simulink model "EMPlanner_cs_old"  (R2020a)
settings: Solver=ode5  StartTime=0.0  StopTime=55  FixedStep=1/1000  RelTol=1e-3
PreLoadFcn:
  | mbxruntime.callbacks.PreLoadFcn(bdroot);
PostLoadFcn:
  | mbxruntime.callbacks.PostLoadFcn(bdroot);
InitFcn:
  | mbxruntime.callbacks.InitFcn(bdroot);
StartFcn:
  | mbxruntime.callbacks.StartFcn(bdroot);
StopFcn:
  | mbxruntime.callbacks.StopFcn(bdroot);
model workspace: external: MAT-File .\EMPlanner_cs_hws.mat (data not in the file)
values from neighbouring files (symbols this model uses):
  c_factor = 43.75    [emplanner_init.m]
  cf = -175016    [emplanner_init.m]
  cr = -130634    [emplanner_init.m]
  KD_PID_distance = 0.0    (= 0)    [emplanner_init.m]
  KD_PID_speed = 0    [emplanner_init.m]
  KI_PID_distance = 0.0    (= 0)    [emplanner_init.m]
  KI_PID_speed = 0    [emplanner_init.m]
  KP_PID_distance = 0.5    [emplanner_init.m]
  KP_PID_speed = 1.8    [emplanner_init.m]
  la = 1.265    [emplanner_init.m]
  lb = 2.947-1.265    (= 1.682)    [emplanner_init.m]
  LQR_K1 = k(:,1)'    [emplanner_init.m]
  LQR_K2 = k(:,2)'    [emplanner_init.m]
  LQR_K3 = k(:,3)'    [emplanner_init.m]
  LQR_K4 = k(:,4)'    [emplanner_init.m]
  m = 2020    [emplanner_init.m]
  path_x = [7.7742 8.77358225507 9.77170536558 10.7685522493 11.7641171228 12.7583983581 13.7513958557 14.7431100776 15.7335416918 16.7226914411 17.7105600952 18.6971484329 ... (551 elements, 551x1)]    [test_path.mat]
  path_y = [-207.8202 -207.82020006 -207.820200616 -207.820202023 -207.82020429 -207.820207237 -207.820210603 -207.820214131 -207.82021762 -207.820220941 -207.820224011 -207.820226778 ... (551 elements, 551x1)]    [test_path.mat]
  rack_displacement = [-39.14 , -37.2 , -35.29 , -33.43 , -31.6 , -29.81 , -28.06 , -26.34 , -24.66 ,      -23.01 , -21.38 , -19.79 , -18.23 , -16.69 , -15.18 , -13.7 , -12.23 , -10.8 , -9.38 , -7.98 ,     -6.61 , -5.25 , -3.91 , -2.59 , -1.29 , 0 , 1.27 , 2.54 , 3.78 , 5.02 , 6.24 , 7.46 , 8.66 ,      9.86 , 11.05 , 12.24 , 13.41 , 14.59 , 15.76 , 16.92 , 18.09 , 19.25 , 20.42 , 21.59 , 22.76 ,      23.93 , 25.11 , 26 ...(+26 chars)    [emplanner_init.m]
  right_wheel_ground = [-70 ,-67.2 , -64.4 , -61.6 , -58.8 , -56 , -53.2 , -50.4 , -47.6 , -44.8 , -42 ,      -39.2 , -36.4 , -33.6 , -30.8 , -28 , -25.2 , -22.4 , -19.6 , -16.8 , -14 , -11.2 , -8.4 , -5.6 ,      -2.8 , 0 , 2.8 , 5.6 , 8.4 , 11.2 , 14 , 16.8 , 19.6 , 22.4 , 25.2 , 28 , 30.8 , 33.6 , 36.4 ,      39.2 , 42 , 44.8 , 47.6 , 50.4 , 53.2 , 56 , 58.8 , 61.6 , 64.4 , 67.2 , 70 ]    [emplanner_init.m]
  vx_break_point = zeros(1,5000)    [emplanner_init.m]
undefined symbols (not defined in the file or in its folder): aubr, DiscIntNeverNeededParam, tablebr, vubr, warningInitialVelocity, x0
libraries: simulink x19, PreScanSimulinkLibrary x10, simulink_extras x5, Solver_SF x1
(part 7 of 8)

== matlab function EMPlanner_cs_old/Audi_A8_Sedan_1/decision&planning module/EM Planner/calc plan start info and stitch trajectory1 ==
  data: pre_trajectory_x input; plan_start_x output; pre_trajectory_y input; pre_trajectory_heading input; pre_trajectory_kappa input; pre_trajectory_velocity input; pre_trajectory_accel input; pre_trajectory_time input; current_time input; host_x input; host_y input; host_heading_xy input; host_vx input; host_vy input; host_ax input; host_ay input; plan_start_y output; plan_start_heading output; plan_start_kappa output; plan_start_vx output; plan_start_vy output; plan_start_ax output; plan_start_ay output; plan_start_time output; stitch_x output; stitch_y output; stitch_heading output; stitch_kappa output; stitch_speed output; stitch_accel output; stitch_time output
function [plan_start_x,plan_start_y,plan_start_heading,plan_start_kappa,plan_start_vx,plan_start_vy,plan_start_ax,...
    plan_start_ay,plan_start_time,stitch_x,stitch_y,stitch_heading,stitch_kappa,stitch_speed,stitch_accel,stitch_time] ...
    = fcn(pre_trajectory_x,pre_trajectory_y,pre_trajectory_heading,pre_trajectory_kappa,pre_trajectory_velocity,...
    pre_trajectory_accel,pre_trajectory_time,current_time,host_x,host_y,host_heading_xy,host_vx,host_vy,host_ax,host_ay)
%该函数将计算规划的起点以及拼接轨迹的信息
%输入 上一周期的规划结果信息pre_trajectory x ,y,heading,kappa,velocity,accel,time
%     本周期的绝对时间current_time
%     定位信息host x,y,heading,kappa,vx,vy,ax,ay
%输出 规划起点信息plan_start x,y,heading,kappa,vx,vy,ax,ay(vx,vy,ax,ay)是世界坐标系的
%     待拼接的轨迹信息，一般在上一周期的轨迹中的current_time+100ms，往前取20个点。
%     当规划完成后，本周期的规划结果和stitch_trajectory一起拼好发给控制

%输出初始化
stitch_x = zeros(20,1);
stitch_y = zeros(20,1);
stitch_heading = zeros(20,1);
stitch_kappa = zeros(20,1);
stitch_speed = zeros(20,1);
stitch_accel = zeros(20,1);
%时间为负代表没有对应的拼接轨迹
stitch_time = ones(20,1)*-1;

%申明全局变量
persistent is_first_run;
if isempty(is_first_run)
    %代表代码首次运行
    is_first_run = 0;
    %按照轨迹拼接算法，应该用车辆动力学递推，但是首次运行车辆的速度都是0，所以没必要递推了
    plan_start_x = host_x;
    plan_start_y = host_y;
    plan_start_heading = host_heading_xy;
    plan_start_kappa = 0;
    plan_start_vx = 0;
    plan_start_vy = 0;
    plan_start_ax = 0;
    plan_start_ay = 0;
    %规划的起点的时间应该是当前时间+100ms
    plan_start_time = current_time + 0.1;
else
    %该函数不是首次运行
    x_cur = host_x;
    y_cur = host_y;
    heading_cur = host_heading_xy;
    kappa_cur = 0;
    %vx vy ax ay要转换成世界坐标系
    vx_cur = host_vx*cos(heading_cur) - host_vy*sin(heading_cur);
    vy_cur = host_vx*sin(heading_cur) + host_vy*cos(heading_cur);
    ax_cur = host_ax*cos(heading_cur) - host_ay*sin(heading_cur);
    ay_cur = host_ax*sin(heading_cur) + host_ay*cos(heading_cur);
    %规划周期
    dt = 0.1;
    %由于不是首次运行了，有上一时刻的轨迹了，找到上一周期轨迹规划的本周期车辆应该在的位置
    for i = 1:length(pre_trajectory_time) - 1
        if (pre_trajectory_time(i) <= current_time && pre_trajectory_time(i + 1) > current_time)
            break;
        end
    end
    %上一周期规划的本周期的车应该在的位置
    pre_x_desire = pre_trajectory_x(i);
    pre_y_desire = pre_trajectory_y(i);
    pre_heading_desire = pre_trajectory_heading(i);
    %计算横纵向误差
    %切向量
    tor = [cos(pre_heading_desire);sin(pre_heading_desire)];
    %法向量
    nor = [-sin(pre_heading_desire);cos(pre_heading_desire)];
    %误差向量
    d_err = [host_x;host_y] - [pre_x_desire;pre_y_desire];
    %纵向误差
    lon_err = abs(d_err'*tor);
    %横向误差
    lat_err = abs(d_err'*nor);
    %纵向误差大于2.5 横向误差大于0.5 认为控制没跟上
    if (lon_err > 2.5)||(lat_err > 0.5)
        %此分支处理控制未跟上的情况，规划起点通过运动学递推
        plan_start_x = x_cur + vx_cur * dt + 0.5 * ax_cur * dt * dt;
        plan_start_y = y_cur + vy_cur * dt + 0.5 * ay_cur * dt * dt;
        plan_start_vx = vx_cur + ax_cur * dt;
        plan_start_vy = vy_cur + ay_cur * dt;
        plan_start_heading = atan2(plan_start_vy,plan_start_vx);
        plan_start_ax = ax_cur;
        plan_start_ay = ay_cur;
        plan_start_kappa = kappa_cur;
        plan_start_time = current_time + 0.1;
        return;
    else
        %此分支表示控制能跟的上规划，开始拼接
        for j = i:length(pre_trajectory_time) - 1
            if (pre_trajectory_time(j) <= current_time + 0.1)&&(pre_trajectory_time(j + 1) > current_time + 0.1)
                break;
            end
        end
        %注：此算法要能运行需要trajectory的点有很高的密度
        plan_start_x = pre_trajectory_x(j);
        plan_start_y = pre_trajectory_y(j);
        plan_start_heading = pre_trajectory_heading(j);
        plan_start_kappa = pre_trajectory_kappa(j);
        %这里的pre_trajectory的速度,加速度是指轨迹的切向速度，切向加速度
        plan_start_vx = pre_trajectory_velocity(j) * cos(plan_start_heading);
        plan_start_vy = pre_trajectory_velocity(j) * sin(plan_start_heading);
        %pre_trajectory的加速度是切向加速度，要想计算ax,ay还要计算法向加速度
        %计算轨迹在current_time + 100ms 这个点的切向量法向量
        tor = [cos(plan_start_heading);sin(plan_start_heading)];
        nor = [-sin(plan_start_heading);cos(plan_start_heading)];
        a_tor = pre_trajectory_accel(j) * tor;
        a_nor = pre_trajectory_velocity(j)^2 * plan_start_kappa * nor ;
        plan_start_ax = a_tor(1) + a_nor(1);
        plan_start_ay = a_tor(2) + a_nor(2);
        plan_start_time = pre_trajectory_time(j);
        %计算拼接轨迹
        %j 表示 current_time + 0.1 的时间点在 pre_trajectory_time的编号
        %拼接是往从j开始，往前拼接20个，也就是pre_trajectory(j-1),j-2,j-3,....j-19
        %分两种情况，如果j小于20，意味着前面的轨迹点不够20个
        %如果j >= 20,意味着前面的点多于20个
        %还有一个细节需要考虑，pre_trajectory x(j) y(j) ....是规划的起点，那么在轨迹拼接时
        %需不需要在stitch_trajectory中把pre_trajectory x(j) y(j) ....包含进去
        %答案是否定的，不应该包进去，因为规划的起点会在规划模块计算完成后的结果中包含，如果在拼接的时候
        %还要包含，那就等于规划起点包含了两次
        %除非本周期计算的轨迹不包含规划起点，那么stitch_trajectory可以包含规划起点。
        %如果本周期计算的轨迹包含规划起点，那么stitch_trajectory就不可以包含规划起点。
        %我们选择规划包含起点，拼接不包含起点的做法
        
        %把起点去掉
        j = j - 1;
        if j >= 20
            stitch_x = pre_trajectory_x(j - 19:j);
            stitch_y = pre_trajectory_y(j - 19:j);
            stitch_heading = pre_trajectory_heading(j - 19:j);
            stitch_kappa = pre_trajectory_kappa(j - 19:j);
            stitch_speed = pre_trajectory_velocity(j - 19:j);
            stitch_accel = pre_trajectory_accel(j - 19:j);
            stitch_time = pre_trajectory_time(j - 19:j);
        else
            stitch_x(20 - j + 1:20) = pre_trajectory_x(1:j);
            stitch_y(20 - j + 1:20) = pre_trajectory_y(1:j);
            stitch_heading(20 - j + 1:20) = pre_trajectory_heading(1:j);
            stitch_kappa(20 - j + 1:20) = pre_trajectory_kappa(1:j);
            stitch_speed(20 - j + 1:20) = pre_trajectory_velocity(1:j);
            stitch_accel(20 - j + 1:20) = pre_trajectory_accel(1:j);
            stitch_time(20 - j + 1:20) = pre_trajectory_time(1:j);           
        end   
    end    
end

== matlab function EMPlanner_cs_old/Audi_A8_Sedan_1/decision&planning module/EM Planner/genrate index to s ==
  data: path_x_set_gcs input; matchPoint_index_s_set_fcs output; path_y_set_gcs input; path_heading_set_gcs input; origin_match_point_index input; origin_point_x_gcs input; origin_point_y_gcs input
function matchPoint_index_s_set_fcs = fun(path_x_set_gcs,path_y_set_gcs,path_heading_set_gcs,...
    origin_match_point_index,origin_point_x_gcs,origin_point_y_gcs)
% 该函数将以给定路径采样点为s轴 取自身在给定路径上投影点作为坐标原点 来求出每个采样点编号和对应s坐标的集合
% path_x_set_gcs,path_y_set_gcs 给定路径采样点集合
% origin_match_point_index,origin_point_x_gcs,origin_point_y_gcs   坐标原点信息
% 输出初始化
matchPoint_index_s_set_fcs = zeros(length(path_x_set_gcs),1);
% 首先给定路径采样点每个点到第一个采样点的弧长
for i = 2:length(path_x_set_gcs)
    dis = sqrt((path_x_set_gcs(i)-path_x_set_gcs(i-1))^2+(path_y_set_gcs(i)-path_y_set_gcs(i-1))^2); % 以直线代替相邻点弧长
    matchPoint_index_s_set_fcs(i) = dis + matchPoint_index_s_set_fcs(i-1); % 累加得到
end
%再求出坐标原点到第一个采样点的弧长
s = CalSFromOriginPoint(matchPoint_index_s_set_fcs,path_x_set_gcs,path_y_set_gcs,path_heading_set_gcs,...
                            origin_point_x_gcs,origin_point_y_gcs,origin_match_point_index);
% 得到每个采样点到坐标原点的弧长对应关系 亦即真正的s坐标对应编号关系
matchPoint_index_s_set_fcs = matchPoint_index_s_set_fcs - ones(length(path_x_set_gcs),1)*s;
end

== stateflow chart EMPlanner_cs_old/Audi_A8_Sedan_1/Chart ==
  (default) -> (junction 5)
  (junction 5) -> (junction 7)
  (junction 7) -> (junction 9) [order 1] : [i >= 100]
  (junction 7) -> (junction 13) [order 2] : {
      | i = i + 1;
      | }
  (junction 9) -> (junction 11) : {
      | do_planning;
      | i = 1;
      | }
  (junction 11) -> (junction 13)
  (junction 13) -> (junction 16)
  (junction 16) -> (junction 18) [order 1] : [j >= 10]
  (junction 16) -> (junction 22) [order 2] : {
      | j = j + 1;
      | }
  (junction 18) -> (junction 20) : {
      | do_control;
      | j = 1;
      | }
  (junction 20) -> (junction 22)
  (junction 22) -> (junction 25)
  data: i local =1; j local =1
  events: do_planning output FUNCTION_CALL_EVENT; do_control output FUNCTION_CALL_EVENT

== matlab function EMPlanner_cs_old/Audi_A8_Sedan_1/decision&planning module/EM Planner/Cartesian2Frenet/MATLAB Function3 ==
  data: l_set input; s_dot_set output; vx_set input; vy_set input; proj_heading_set input; proj_kappa_set input; l_dot_set output; dl_set output
function [s_dot_set,l_dot_set,dl_set] = fcn(l_set,vx_set,vy_set,proj_heading_set,proj_kappa_set)
%该函数将计算frenet坐标系下的s_dot, l_dot, dl/ds
n = 128;
% 输出初始化
s_dot_set = ones(n,1)*nan;
l_dot_set = ones(n,1)*nan;
dl_set = ones(n,1)*nan;

for i = 1 : length(l_set)
    if isnan(l_set(i))
        break;
    end
    v_h = [vx_set(i);vy_set(i)];
    n_r = [-sin(proj_heading_set(i));cos(proj_heading_set(i))];
    t_r = [cos(proj_heading_set(i));sin(proj_heading_set(i))];
    l_dot_set(i) = v_h'*n_r;
    s_dot_set(i) = v_h'*t_r/(1 - proj_kappa_set(i)*l_set(i));
    %%%向量法做cartesian与frenet的转换要更简单，但是也有缺点，向量法必须依赖速度加速度
    %l' = l_dot/s_dot 但是如果s_dot = 0 此方法就失效了
    if abs(s_dot_set(i)) < 1e-6
        dl_set(i) = 0;
    else
        dl_set(i) = l_dot_set(i)/s_dot_set(i);
    end
end

== matlab function EMPlanner_cs_old/Audi_A8_Sedan_1/decision&planning module/EM Planner/Cartesian2Frenet/MATLAB Function ==
  data: x_set_gcs input; s_set_fcs output; y_set_gcs input; path_x_set_gcs input; path_y_set_gcs input; path_heading_set_gcs input; match_point_index_set input; proj_point_x_set_gcs input; proj_point_y_set_gcs input; proj_point_heading_set_gcs input; l_set_fcs output; matchPoint_index_s_set_fcs input
function [s_set_fcs,l_set_fcs] = fun(x_set_gcs,y_set_gcs,path_x_set_gcs,path_y_set_gcs,path_heading_set_gcs,match_point_index_set,...
    proj_point_x_set_gcs,proj_point_y_set_gcs,proj_point_heading_set_gcs,matchPoint_index_s_set_fcs)
% 将函数批量将给定点的(x,y)转化成(s,l)
% 假设最多有181个点需要转换坐标
n = 181;
% 输出初始化
s_set_fcs = ones(n,1)*nan; l_set_fcs = ones(n,1)*nan;
for i = 1:length(x_set_gcs)
    if isnan(x_set_gcs(i))
        break;
    end
    s_set_fcs(i) = CalSFromOriginPoint(matchPoint_index_s_set_fcs,path_x_set_gcs,path_y_set_gcs,path_heading_set_gcs,...
                                proj_point_x_set_gcs(i),proj_point_y_set_gcs(i),match_point_index_set(i));
    vector_rh = [x_set_gcs(i),y_set_gcs(i)];
    vector_rp = [proj_point_x_set_gcs(i),proj_point_y_set_gcs(i)];
    vector_np = [-sin(proj_point_heading_set_gcs(i)),cos(proj_point_heading_set_gcs(i))];
    l_set_fcs(i) = dot(vector_rh-vector_rp, vector_np);
end
end

== matlab function EMPlanner_cs_old/Audi_A8_Sedan_2/PathFollower_Preview_1/LateralController/Calculate delta steering error/eml_delta_steering_error ==
  data: v_x_vehicle input; v_x_vehicle_Min input; t_Preview_LatCtrl input; delta_steeringwheeltotal output; v_y_vehicle input; yawrate_vehicle input; CorneringStiffness_Tyres_Front input; CorneringStiffness_Tyres_Rear input; m_vehicle_total input; inertia_z_vehicle_total input; e_Lat input size=10; Pos_x_CoG_Vehicle input; wheelbase input; RefreshCounter parameter
function delta_steeringwheeltotal = eml_delta_steering_error(v_x_vehicle,v_x_vehicle_Min,t_Preview_LatCtrl,v_y_vehicle,yawrate_vehicle,CorneringStiffness_Tyres_Front,CorneringStiffness_Tyres_Rear,m_vehicle_total,inertia_z_vehicle_total,e_Lat,Pos_x_CoG_Vehicle,wheelbase,RefreshCounter)

delta_steeringwheeltotal = emlfcn_delta_steering_error(v_x_vehicle,v_x_vehicle_Min,t_Preview_LatCtrl,v_y_vehicle,yawrate_vehicle,CorneringStiffness_Tyres_Front,CorneringStiffness_Tyres_Rear,m_vehicle_total,inertia_z_vehicle_total,e_Lat,Pos_x_CoG_Vehicle,wheelbase,RefreshCounter);

% end function

== matlab function EMPlanner_cs_old/Audi_A8_Sedan_1/decision&planning module/EM Planner/MATLAB Function2 ==
  data: x_set_gcs input; match_point_index_set output; y_set_gcs input; path_x_set_gcs input; path_y_set_gcs input; path_heading_set_gcs input; path_kappa_set_gcs input; proj_point_x_set_gcs output; proj_point_y_set_gcs output; proj_point_heading_set_gcs output; proj_point_kappa_set_gcs output
function [match_point_index_set,proj_point_x_set_gcs,proj_point_y_set_gcs,proj_point_heading_set_gcs,...
    proj_point_kappa_set_gcs] = fcn(x_set_gcs,y_set_gcs,path_x_set_gcs,path_y_set_gcs,...
    path_heading_set_gcs,path_kappa_set_gcs)
% 该函数将批量计算点在给定路径下的匹配点编号和投影点信息   
% x_set_gcs,y_set_gcs 输入点信息集合
% path_x_set_gcs,path_y_set_gcs,path_heading_set_gcs,path_kappa_set_gcs 给定路径点信息集合
% match_point_index_set 匹配点编号集合
% proj_point_x_set_gcs,proj_point_y_set_gcs,proj_point_heading_set_gcs,proj_point_kappa_set_gcs 投影点信息集合

% 假设最多有181个点需要投影
n = 181;
% 对输出进行初始化
match_point_index_set = ones(n,1) *nan; 
proj_point_x_set_gcs = ones(n,1) *nan;  proj_point_y_set_gcs = ones(n,1) *nan;
proj_point_heading_set_gcs = ones(n,1) *nan;  proj_point_kappa_set_gcs = ones(n,1) *nan;

% 寻找匹配点时 需要利用上一个周期的结果 因此定义需要利用的静态变量
persistent is_first_run;
persistent pre_match_point_index_set;
persistent pre_path_x_set_gcs; persistent pre_path_y_set_gcs; % 通过上个周期匹配点位矢判断遍历方向
persistent pre_path_heading_set_gcs; persistent pre_path_kappa_set_gcs;
persistent pre_x_set_gcs; persistent pre_y_set_gcs; % 判断相邻帧检测的是否是同一个障碍物

if isempty(is_first_run)
    is_first_run = 0;
    % 首次运行 所有待求点都从给定路径路径第一个点开始找 往前遍历 且距离连续增长上限设为50
    for i = 1:length(x_set_gcs) % 存在的点都在前面 遍历到nan至后面的点都不存在
        if isnan(x_set_gcs(i))
            break;
        end
        start_find_index = 1; forward_stable_backward = 1; increase_count_limit = 50;
        % 计算匹配点编号
        match_point_index = CalMatchPointIndex(x_set_gcs(i),y_set_gcs(i),path_x_set_gcs,...
        path_y_set_gcs,path_heading_set_gcs,path_kappa_set_gcs,start_find_index,...
        increase_count_limit, forward_stable_backward);
        % 计算投影点信息
        [proj_point_x_gcs,proj_point_y_gcs,proj_point_heading_gcs,proj_point_kappa_gcs] = ...
        CalProjPointInfo(x_set_gcs(i),y_set_gcs(i),path_x_set_gcs,path_y_set_gcs,path_heading_set_gcs,...
        path_kappa_set_gcs,match_point_index);
        % 将每个点求解信息添加到集合
        match_point_index_set(i) = match_point_index;
        proj_point_x_set_gcs(i) = proj_point_x_gcs; proj_point_y_set_gcs(i) = proj_point_y_gcs;
        proj_point_heading_set_gcs(i) = proj_point_heading_gcs; 
        proj_point_kappa_set_gcs(i) = proj_point_kappa_gcs;
    end
    % 保存该周期信息 以便下周期使用
    pre_match_point_index_set = match_point_index_set;
    pre_path_x_set_gcs = path_x_set_gcs; pre_path_y_set_gcs = path_y_set_gcs;
    pre_path_heading_set_gcs = path_heading_set_gcs; pre_path_kappa_set_gcs = path_kappa_set_gcs;
    pre_x_set_gcs = x_set_gcs; pre_y_set_gcs = y_set_gcs;
else
    % 需要使用上周期信息
    for i = 1:length(x_set_gcs)
        if isnan(x_set_gcs(i))
            break;
        end
        % 检测相邻帧是否是同一物体求解
        dis = sqrt((x_set_gcs(i)-pre_x_set_gcs(i))^2 + (y_set_gcs(i)-pre_y_set_gcs(i))^2);
        if dis > 10  % 相邻帧(相隔0.1s)同一物体距离不可能这么大
            % 说明相邻帧不是同一物体 上周期该物体已经消失在车辆的检测范围内
            % 把上周期该物体匹配点编号信息清空
            pre_match_point_index_set(i) = nan;
        end
        if isnan(pre_match_point_index_set(i))
            % 说明该物体是第一次寻找匹配点 从头开始寻找 且往前遍历
            start_find_index = 1; forward_stable_backward = 1; increase_count_limit = 50;
        else
            % 说明该物体上周期已经寻找过匹配点  判断开始寻找编号 和遍历方向
            start_find_index = pre_match_point_index_set(i); increase_count_limit = 5;
            % 提取上周期匹配点信息
            pre_match_point_x = pre_path_x_set_gcs(pre_match_point_index_set(i));
            pre_match_point_y = pre_path_y_set_gcs(pre_match_point_index_set(i));
            pre_match_point_heading = pre_path_heading_set_gcs(pre_match_point_index_set(i));
            % 通过该物体上周期匹配点位置到本周期位置向量和上周期匹配点切向量的点乘来判断遍历方向
            vector_preMatch_current = [x_set_gcs(i),y_set_gcs(i)] - [pre_match_point_x, pre_match_point_y];
            vector_tor_preMatch = [cos(pre_match_point_heading), sin(pre_match_point_heading)];
            forward_stable_backward = dot(vector_preMatch_current, vector_tor_preMatch);
        end
        % 计算匹配点编号
        match_point_index = CalMatchPointIndex(x_set_gcs(i),y_set_gcs(i),path_x_set_gcs,...
        path_y_set_gcs,path_heading_set_gcs,path_kappa_set_gcs,start_find_index,...
        increase_count_limit, forward_stable_backward);
        % 计算投影点信息
        [proj_point_x_gcs,proj_point_y_gcs,proj_point_heading_gcs,proj_point_kappa_gcs] = ...
        CalProjPointInfo(x_set_gcs(i),y_set_gcs(i),path_x_set_gcs,path_y_set_gcs,path_heading_set_gcs,...
        path_kappa_set_gcs,match_point_index);
        % 将每个点求解信息添加到集合
        match_point_index_set(i) = match_point_index;
        proj_point_x_set_gcs(i) = proj_point_x_gcs; proj_point_y_set_gcs(i) = proj_point_y_gcs;
        proj_point_heading_set_gcs(i) = proj_point_heading_gcs; 
        proj_point_kappa_set_gcs(i) = proj_point_kappa_gcs;
    end
    % 保存该周期信息 以便下周期使用
    pre_match_point_index_set = match_point_index_set;
    pre_path_x_set_gcs = path_x_set_gcs; pre_path_y_set_gcs = path_y_set_gcs;
    pre_path_heading_set_gcs = path_heading_set_gcs; pre_path_kappa_set_gcs = path_kappa_set_gcs;
    pre_x_set_gcs = x_set_gcs; pre_y_set_gcs = y_set_gcs;
end
end

== matlab function EMPlanner_cs_old/Audi_A8_Sedan_1/decision&planning module/EM Planner/Cartesian2Frenet/MATLAB Function4 ==
  data: ax_set input; s_dot2_set output; ay_set input; proj_heading_set input; proj_kappa_set input; l_set input; s_dot_set input; dl_set input; l_dot2_set output; ddl_set output
function [s_dot2_set,l_dot2_set,ddl_set] = fcn(ax_set,ay_set,proj_heading_set,proj_kappa_set,l_set,s_dot_set,dl_set)
%由于不知道有多少个点需要做坐标转换，设一个最大值做缓冲
n = 128;
% 输出初始化
s_dot2_set = ones(n,1)*nan;
l_dot2_set = ones(n,1)*nan;
ddl_set = ones(n,1)*nan;

for i = 1:length(l_set)
    if isnan(l_set(i))
       break;
    end
    a_h = [ax_set(i);ay_set(i)];
    n_r = [-sin(proj_heading_set(i));cos(proj_heading_set(i))];
    t_r = [cos(proj_heading_set(i));sin(proj_heading_set(i))];
    %近似认为dkr/ds 为0 简化计算
    l_dot2_set(i) = a_h'*n_r - proj_kappa_set(i) * (1 - proj_kappa_set(i) * l_set(i)) * s_dot_set(i)^2;
    s_dot2_set(i) = (1/(1 - proj_kappa_set(i) * l_set(i)))* (a_h' * t_r + 2 * proj_kappa_set(i) * dl_set(i) * s_dot_set(i)^2);
    % 要考虑加速度为0的情况
    if (s_dot2_set(i) < 1e-6)
        ddl_set(i) = 0;
    else
        ddl_set(i) = (l_dot2_set(i) - dl_set(i)*s_dot2_set(i))/(s_dot_set(i)^2);
    end
end

== matlab function EMPlanner_cs_old/Audi_A8_Sedan_1/decision&planning module/EM Planner/increase DP path nodes1 ==
  data: plan_start_point_s_fcs input; dp_path_s_final_set_fcs output; plan_start_point_l_fcs input; plan_start_point_dl_fcs input; plan_start_point_ddl_fcs input; dp_path_s_init_set_fcs input; dp_path_l_init_set_fcs input; dp_path_l_final_set_fcs output; dp_path_dl_final_set_fcs output; dp_path_ddl_final_set_fcs output
function [dp_path_s_final_set_fcs,dp_path_l_final_set_fcs,dp_path_dl_final_set_fcs,dp_path_ddl_final_set_fcs] = ...
    fcn(plan_start_point_s_fcs,plan_start_point_l_fcs,plan_start_point_dl_fcs,plan_start_point_ddl_fcs,dp_path_s_init_set_fcs,dp_path_l_init_set_fcs)
% 原有的动态规划的路径点太少  该函数用来增密路径点
% 输入:plan_start_point_info_fcs 规划起点信息 dp_path_info_init_set_fcs 动态规划初始点集合信息
% 输出:dp_path_info_final_set_fcs 动态规划最终点集合信息
% 原有的动态规划的路径点太少  该函数用来增密原有的动态规划得到的初始路径点
% 通过原有的规划点进行增密
% 假设增密之后横向每隔一米踩一个点
ds = 1;
% 原来路径为 规划起点-> 动态规划点1 -> 动态规划点2 -> 动态规划点3 -> 动态规划点4 -> 动态规划点5
% 增密后路径为 规划起点->(新增点->新增点->新增点)->动态规划点1->(新增点->新增点->新增点)->动态规划点2->...
% 如 规划起点-> 动态规划点1 为一个五次多项式  通过ds取多项式多个点 即为新增的点

% 假设增密之后最多200个点
n = 200;
% 输出初始化
dp_path_s_final_set_fcs = ones(n,1)*nan;dp_path_l_final_set_fcs = ones(n,1)*nan;
dp_path_dl_final_set_fcs = ones(n,1)*nan; dp_path_ddl_final_set_fcs = ones(n,1)*nan;

% 第一个五次多项式的起点为规划起点
start_s = plan_start_point_s_fcs; start_l = plan_start_point_l_fcs; 
start_dl = plan_start_point_dl_fcs; start_ddl = plan_start_point_ddl_fcs;

s_cur = []; l_cur = []; dl_cur = []; ddl_cur = []; %开辟动态数组存储所有采样点

for i = 1:length(dp_path_s_init_set_fcs)
    if isnan(dp_path_s_init_set_fcs(i))
        break;   %点不存在 退出
    end
    s_temp = []; l_temp = []; dl_temp = []; ddl_temp = []; %开辟临时动态数组存储当前循环采样点
    % 对规划起点-> 动态规划点1 -> 动态规划点2 -> 动态规划点3 -> 动态规划点4 -> 动态规划点5->...进行采样
    for j = 1:10000  % 取个较大的循环 下面通过条件break退出循环就
        s_node = start_s + ds * (j-1);   %增密后各个采样点s坐标  l,dl,ddl需要通过五次多项式计算
        if s_node < dp_path_s_init_set_fcs(i)
            s_temp = [s_temp, s_node]; % 将满足条件的增密点添加进数组
        else
            break;
        end
    end
    % % 求出五次多项式终点的边界条件
    end_s = dp_path_s_init_set_fcs(i); end_l = dp_path_l_init_set_fcs(i); end_dl = 0; end_ddl = 0;
    [a0,a1,a2,a3,a4,a5] = CalQuinticCoeffient(start_s,start_l,start_dl,start_ddl,end_s,end_l,end_dl,end_ddl);
    % 通过五次多项式求出每个采样点的l,dl,ddl
    for k = 1:length(s_temp)
        l_node = a0 + a1 * s_temp(k) + a2 * s_temp(k)^2+ a3 * s_temp(k)^3 + a4 * s_temp(k)^4 + a5 * s_temp(k)^5;
        l_temp = [l_temp,l_node];
        dl_node = a1 + 2 * a2 * s_temp(k) + 3 * a3 * s_temp(k)^2 + 4 * a4 * s_temp(k)^3 + 5 * a5 * s_temp(k)^4;
        dl_temp = [dl_temp,dl_node];
        ddl_node = 2 * a2 + 6 * a3 * s_temp(k) + 12 * a4 * s_temp(k)^2 + 20 * a5 * s_temp(k)^3;
        ddl_temp = [ddl_temp, ddl_node];
    end 
    % 将当前循环记录的采样点信息记录到总的动态数组里
    s_cur = [s_cur, s_temp]; l_cur = [l_cur, l_temp]; dl_cur = [dl_cur, dl_temp]; ddl_cur = [ddl_cur, ddl_temp];           
     % end的值赋值给start 做下一步循环
    start_s = end_s;start_l = end_l;start_dl = end_dl;start_ddl = end_ddl;
end

for i = 1:length(s_cur)
    % 防止增密之后点的个数超过最大容量
    if i > n
        break;
    end
    % 保证s坐标严格单调上升
    dp_path_s_final_set_fcs(i) = plan_start_point_s_fcs + ds * (i - 1);
%     dp_path_s_final_set_fcs(i) = s_cur(i);
    dp_path_l_final_set_fcs(i) = l_cur(i);
    dp_path_dl_final_set_fcs(i) = dl_cur(i);
    dp_path_ddl_final_set_fcs(i) = ddl_cur(i);
end
end

== matlab function EMPlanner_cs_old/Audi_A8_Sedan_1/decision&planning module/EM Planner/obs/MATLAB Function3 ==
  data: x_set_gcs input; match_point_index_set output; y_set_gcs input; path_x_set_gcs input; path_y_set_gcs input; path_heading_set_gcs input; path_kappa_set_gcs input; proj_point_x_set_gcs output; proj_point_y_set_gcs output; proj_point_heading_set_gcs output; proj_point_kappa_set_gcs output
function [match_point_index_set,proj_point_x_set_gcs,proj_point_y_set_gcs,proj_point_heading_set_gcs,...
    proj_point_kappa_set_gcs] = fcn(x_set_gcs,y_set_gcs,path_x_set_gcs,path_y_set_gcs,...
    path_heading_set_gcs,path_kappa_set_gcs)
% 该函数将批量计算点在给定路径下的匹配点编号和投影点信息   
% x_set_gcs,y_set_gcs 输入点信息集合
% path_x_set_gcs,path_y_set_gcs,path_heading_set_gcs,path_kappa_set_gcs 给定路径点信息集合
% match_point_index_set 匹配点编号集合
% proj_point_x_set_gcs,proj_point_y_set_gcs,proj_point_heading_set_gcs,proj_point_kappa_set_gcs 投影点信息集合

% 假设最多有181个点需要投影
n = 181;
% 对输出进行初始化
match_point_index_set = ones(n,1) *nan; 
proj_point_x_set_gcs = ones(n,1) *nan;  proj_point_y_set_gcs = ones(n,1) *nan;
proj_point_heading_set_gcs = ones(n,1) *nan;  proj_point_kappa_set_gcs = ones(n,1) *nan;

% 寻找匹配点时 需要利用上一个周期的结果 因此定义需要利用的静态变量
persistent is_first_run;
persistent pre_match_point_index_set;
persistent pre_path_x_set_gcs; persistent pre_path_y_set_gcs; % 通过上个周期匹配点位矢判断遍历方向
persistent pre_path_heading_set_gcs; persistent pre_path_kappa_set_gcs;
persistent pre_x_set_gcs; persistent pre_y_set_gcs; % 判断相邻帧检测的是否是同一个障碍物

if isempty(is_first_run)
    is_first_run = 0;
    % 首次运行 所有待求点都从给定路径路径第一个点开始找 往前遍历 且距离连续增长上限设为50
    for i = 1:length(x_set_gcs) % 存在的点都在前面 遍历到nan至后面的点都不存在
        if isnan(x_set_gcs(i))
            break;
        end
        start_find_index = 1; forward_stable_backward = 1; increase_count_limit = 50;
        % 计算匹配点编号
        match_point_index = CalMatchPointIndex(x_set_gcs(i),y_set_gcs(i),path_x_set_gcs,...
        path_y_set_gcs,path_heading_set_gcs,path_kappa_set_gcs,start_find_index,...
        increase_count_limit, forward_stable_backward);
        % 计算投影点信息
        [proj_point_x_gcs,proj_point_y_gcs,proj_point_heading_gcs,proj_point_kappa_gcs] = ...
        CalProjPointInfo(x_set_gcs(i),y_set_gcs(i),path_x_set_gcs,path_y_set_gcs,path_heading_set_gcs,...
        path_kappa_set_gcs,match_point_index);
        % 将每个点求解信息添加到集合
        match_point_index_set(i) = match_point_index;
        proj_point_x_set_gcs(i) = proj_point_x_gcs; proj_point_y_set_gcs(i) = proj_point_y_gcs;
        proj_point_heading_set_gcs(i) = proj_point_heading_gcs; 
        proj_point_kappa_set_gcs(i) = proj_point_kappa_gcs;
    end
    % 保存该周期信息 以便下周期使用
    pre_match_point_index_set = match_point_index_set;
    pre_path_x_set_gcs = path_x_set_gcs; pre_path_y_set_gcs = path_y_set_gcs;
    pre_path_heading_set_gcs = path_heading_set_gcs; pre_path_kappa_set_gcs = path_kappa_set_gcs;
    pre_x_set_gcs = x_set_gcs; pre_y_set_gcs = y_set_gcs;
else
    % 需要使用上周期信息
    for i = 1:length(x_set_gcs)
        if isnan(x_set_gcs(i))
            break;
        end
        % 检测相邻帧是否是同一物体求解
        dis = sqrt((x_set_gcs(i)-pre_x_set_gcs(i))^2 + (y_set_gcs(i)-pre_y_set_gcs(i))^2);
        if dis > 10  % 相邻帧(相隔0.1s)同一物体距离不可能这么大
            % 说明相邻帧不是同一物体 上周期该物体已经消失在车辆的检测范围内
            % 把上周期该物体匹配点编号信息清空
            pre_match_point_index_set(i) = nan;
        end
        if isnan(pre_match_point_index_set(i))
            % 说明该物体是第一次寻找匹配点 从头开始寻找 且往前遍历
            start_find_index = 1; forward_stable_backward = 1; increase_count_limit = 50;
        else
            % 说明该物体上周期已经寻找过匹配点  判断开始寻找编号 和遍历方向
            start_find_index = pre_match_point_index_set(i); increase_count_limit = 5;
            % 提取上周期匹配点信息
            pre_match_point_x = pre_path_x_set_gcs(pre_match_point_index_set(i));
            pre_match_point_y = pre_path_y_set_gcs(pre_match_point_index_set(i));
            pre_match_point_heading = pre_path_heading_set_gcs(pre_match_point_index_set(i));
            % 通过该物体上周期匹配点位置到本周期位置向量和上周期匹配点切向量的点乘来判断遍历方向
            vector_preMatch_current = [x_set_gcs(i),y_set_gcs(i)] - [pre_match_point_x, pre_match_point_y];
            vector_tor_preMatch = [cos(pre_match_point_heading), sin(pre_match_point_heading)];
            forward_stable_backward = dot(vector_preMatch_current, vector_tor_preMatch);
        end
        % 计算匹配点编号
        match_point_index = CalMatchPointIndex(x_set_gcs(i),y_set_gcs(i),path_x_set_gcs,...
        path_y_set_gcs,path_heading_set_gcs,path_kappa_set_gcs,start_find_index,...
        increase_count_limit, forward_stable_backward);
        % 计算投影点信息
        [proj_point_x_gcs,proj_point_y_gcs,proj_point_heading_gcs,proj_point_kappa_gcs] = ...
        CalProjPointInfo(x_set_gcs(i),y_set_gcs(i),path_x_set_gcs,path_y_set_gcs,path_heading_set_gcs,...
        path_kappa_set_gcs,match_point_index);
        % 将每个点求解信息添加到集合
        match_point_index_set(i) = match_point_index;
        proj_point_x_set_gcs(i) = proj_point_x_gcs; proj_point_y_set_gcs(i) = proj_point_y_gcs;
        proj_point_heading_set_gcs(i) = proj_point_heading_gcs; 
        proj_point_kappa_set_gcs(i) = proj_point_kappa_gcs;
    end
    % 保存该周期信息 以便下周期使用
    pre_match_point_index_set = match_point_index_set;
    pre_path_x_set_gcs = path_x_set_gcs; pre_path_y_set_gcs = path_y_set_gcs;
    pre_path_heading_set_gcs = path_heading_set_gcs; pre_path_kappa_set_gcs = path_kappa_set_gcs;
    pre_x_set_gcs = x_set_gcs; pre_y_set_gcs = y_set_gcs;
end
end

== matlab function EMPlanner_cs_old/Audi_A8_Sedan_1/decision&planning module/EM Planner/obs/Cartesian2Frenet1/MATLAB Function ==
  data: x_set_gcs input; s_set_fcs output; y_set_gcs input; path_x_set_gcs input; path_y_set_gcs input; path_heading_set_gcs input; match_point_index_set input; proj_point_x_set_gcs input; proj_point_y_set_gcs input; proj_point_heading_set_gcs input; l_set_fcs output; matchPoint_index_s_set_fcs input
function [s_set_fcs,l_set_fcs] = fun(x_set_gcs,y_set_gcs,path_x_set_gcs,path_y_set_gcs,path_heading_set_gcs,match_point_index_set,...
    proj_point_x_set_gcs,proj_point_y_set_gcs,proj_point_heading_set_gcs,matchPoint_index_s_set_fcs)
% 将函数批量将给定点的(x,y)转化成(s,l)
% 假设最多有181个点需要转换坐标
n = 181;
% 输出初始化
s_set_fcs = ones(n,1)*nan; l_set_fcs = ones(n,1)*nan;
for i = 1:length(x_set_gcs)
    if isnan(x_set_gcs(i))
        break;
    end
    s_set_fcs(i) = CalSFromOriginPoint(matchPoint_index_s_set_fcs,path_x_set_gcs,path_y_set_gcs,path_heading_set_gcs,...
                                proj_point_x_set_gcs(i),proj_point_y_set_gcs(i),match_point_index_set(i));
    vector_rh = [x_set_gcs(i),y_set_gcs(i)];
    vector_rp = [proj_point_x_set_gcs(i),proj_point_y_set_gcs(i)];
    vector_np = [-sin(proj_point_heading_set_gcs(i)),cos(proj_point_heading_set_gcs(i))];
    l_set_fcs(i) = dot(vector_rh-vector_rp, vector_np);
end
end

== matlab function EMPlanner_cs_old/Audi_A8_Sedan_1/decision&planning module/referenceline provider/solve heading and kappa求解给定path的heading角和曲率 ==
  data: path_x_set_gcs output; path_y_set_gcs output; path_heading_set_gcs output; path_x_set_gcs input; path_y_set_gcs input; path_kappa_set_gcs output
function [path_x_set_gcs,path_y_set_gcs,path_heading_set_gcs,path_kappa_set_gcs] = fcn(path_x_set_gcs,path_y_set_gcs)
%该函数将计算全局路径的切线方向与x轴的夹角和曲率
%输入：path_x_set_gcs,path_y_set_gcs 给定路径坐标 都是列向量
%输出：path_heading_gcs path_kappa_gcs 给定路径的heading和曲率
%输出初始化
if isrow(path_x_set_gcs)
    path_x_set_gcs = path_x_set_gcs';   % 保证为列向量
    path_y_set_gcs = path_y_set_gcs';
end
[path_heading_set_gcs,path_kappa_set_gcs] = CalHeadingAndKappa(path_x_set_gcs,path_y_set_gcs);
end

== matlab function EMPlanner_cs_old/Audi_A8_Sedan_1/decision&planning module/referenceline provider/MATLAB Function6 ==
  data: x_set_gcs input; match_point_index_set output; y_set_gcs input; path_x_set_gcs input; path_y_set_gcs input; path_heading_set_gcs input; path_kappa_set_gcs input; proj_point_x_set_gcs output; proj_point_y_set_gcs output; proj_point_heading_set_gcs output; proj_point_kappa_set_gcs output
function [match_point_index_set,proj_point_x_set_gcs,proj_point_y_set_gcs,proj_point_heading_set_gcs,...
    proj_point_kappa_set_gcs] = fcn(x_set_gcs,y_set_gcs,path_x_set_gcs,path_y_set_gcs,...
    path_heading_set_gcs,path_kappa_set_gcs)
% 该函数将批量计算点在给定路径下的匹配点编号和投影点信息   
% x_set_gcs,y_set_gcs 输入点信息集合
% path_x_set_gcs,path_y_set_gcs,path_heading_set_gcs,path_kappa_set_gcs 给定路径点信息集合
% match_point_index_set 匹配点编号集合
% proj_point_x_set_gcs,proj_point_y_set_gcs,proj_point_heading_set_gcs,proj_point_kappa_set_gcs 投影点信息集合

% 假设最多有181个点需要投影
n = 181;
% 对输出进行初始化
match_point_index_set = ones(n,1) *nan; 
proj_point_x_set_gcs = ones(n,1) *nan;  proj_point_y_set_gcs = ones(n,1) *nan;
proj_point_heading_set_gcs = ones(n,1) *nan;  proj_point_kappa_set_gcs = ones(n,1) *nan;

% 寻找匹配点时 需要利用上一个周期的结果 因此定义需要利用的静态变量
persistent is_first_run;
persistent pre_match_point_index_set;
persistent pre_path_x_set_gcs; persistent pre_path_y_set_gcs; % 通过上个周期匹配点位矢判断遍历方向
persistent pre_path_heading_set_gcs; persistent pre_path_kappa_set_gcs;
persistent pre_x_set_gcs; persistent pre_y_set_gcs; % 判断相邻帧检测的是否是同一个障碍物

if isempty(is_first_run)
    is_first_run = 0;
    % 首次运行 所有待求点都从给定路径路径第一个点开始找 往前遍历 且距离连续增长上限设为50
    for i = 1:length(x_set_gcs) % 存在的点都在前面 遍历到nan至后面的点都不存在
        if isnan(x_set_gcs(i))
            break;
        end
        start_find_index = 1; forward_stable_backward = 1; increase_count_limit = 50;
        % 计算匹配点编号
        match_point_index = CalMatchPointIndex(x_set_gcs(i),y_set_gcs(i),path_x_set_gcs,...
        path_y_set_gcs,path_heading_set_gcs,path_kappa_set_gcs,start_find_index,...
        increase_count_limit, forward_stable_backward);
        % 计算投影点信息
        [proj_point_x_gcs,proj_point_y_gcs,proj_point_heading_gcs,proj_point_kappa_gcs] = ...
        CalProjPointInfo(x_set_gcs(i),y_set_gcs(i),path_x_set_gcs,path_y_set_gcs,path_heading_set_gcs,...
        path_kappa_set_gcs,match_point_index);
        % 将每个点求解信息添加到集合
        match_point_index_set(i) = match_point_index;
        proj_point_x_set_gcs(i) = proj_point_x_gcs; proj_point_y_set_gcs(i) = proj_point_y_gcs;
        proj_point_heading_set_gcs(i) = proj_point_heading_gcs; 
        proj_point_kappa_set_gcs(i) = proj_point_kappa_gcs;
    end
    % 保存该周期信息 以便下周期使用
    pre_match_point_index_set = match_point_index_set;
    pre_path_x_set_gcs = path_x_set_gcs; pre_path_y_set_gcs = path_y_set_gcs;
    pre_path_heading_set_gcs = path_heading_set_gcs; pre_path_kappa_set_gcs = path_kappa_set_gcs;
    pre_x_set_gcs = x_set_gcs; pre_y_set_gcs = y_set_gcs;
else
    % 需要使用上周期信息
    for i = 1:length(x_set_gcs)
        if isnan(x_set_gcs(i))
            break;
        end
        % 检测相邻帧是否是同一物体求解
        dis = sqrt((x_set_gcs(i)-pre_x_set_gcs(i))^2 + (y_set_gcs(i)-pre_y_set_gcs(i))^2);
        if dis > 10  % 相邻帧(相隔0.1s)同一物体距离不可能这么大
            % 说明相邻帧不是同一物体 上周期该物体已经消失在车辆的检测范围内
            % 把上周期该物体匹配点编号信息清空
            pre_match_point_index_set(i) = nan;
        end
        if isnan(pre_match_point_index_set(i))
            % 说明该物体是第一次寻找匹配点 从头开始寻找 且往前遍历
            start_find_index = 1; forward_stable_backward = 1; increase_count_limit = 50;
        else
            % 说明该物体上周期已经寻找过匹配点  判断开始寻找编号 和遍历方向
            start_find_index = pre_match_point_index_set(i); increase_count_limit = 5;
            % 提取上周期匹配点信息
            pre_match_point_x = pre_path_x_set_gcs(pre_match_point_index_set(i));
            pre_match_point_y = pre_path_y_set_gcs(pre_match_point_index_set(i));
            pre_match_point_heading = pre_path_heading_set_gcs(pre_match_point_index_set(i));
            % 通过该物体上周期匹配点位置到本周期位置向量和上周期匹配点切向量的点乘来判断遍历方向
            vector_preMatch_current = [x_set_gcs(i),y_set_gcs(i)] - [pre_match_point_x, pre_match_point_y];
            vector_tor_preMatch = [cos(pre_match_point_heading), sin(pre_match_point_heading)];
            forward_stable_backward = dot(vector_preMatch_current, vector_tor_preMatch);
        end
        % 计算匹配点编号
        match_point_index = CalMatchPointIndex(x_set_gcs(i),y_set_gcs(i),path_x_set_gcs,...
        path_y_set_gcs,path_heading_set_gcs,path_kappa_set_gcs,start_find_index,...
        increase_count_limit, forward_stable_backward);
        % 计算投影点信息
        [proj_point_x_gcs,proj_point_y_gcs,proj_point_heading_gcs,proj_point_kappa_gcs] = ...
        CalProjPointInfo(x_set_gcs(i),y_set_gcs(i),path_x_set_gcs,path_y_set_gcs,path_heading_set_gcs,...
        path_kappa_set_gcs,match_point_index);
        % 将每个点求解信息添加到集合
        match_point_index_set(i) = match_point_index;
        proj_point_x_set_gcs(i) = proj_point_x_gcs; proj_point_y_set_gcs(i) = proj_point_y_gcs;
        proj_point_heading_set_gcs(i) = proj_point_heading_gcs; 
        proj_point_kappa_set_gcs(i) = proj_point_kappa_gcs;
    end
    % 保存该周期信息 以便下周期使用
    pre_match_point_index_set = match_point_index_set;
    pre_path_x_set_gcs = path_x_set_gcs; pre_path_y_set_gcs = path_y_set_gcs;
    pre_path_heading_set_gcs = path_heading_set_gcs; pre_path_kappa_set_gcs = path_kappa_set_gcs;
    pre_x_set_gcs = x_set_gcs; pre_y_set_gcs = y_set_gcs;
end
end

== matlab function EMPlanner_cs_old/Audi_A8_Sedan_1/decision&planning module/EM Planner/Cartesian2Frenet/MATLAB Function1 ==
  data: l_set_fcs input; sdot_set_fcs output; vx_set_gcs input; vy_set_gcs input; proj_point_heading_set_gcs input; proj_point_kappa_set_gcs input; ldot_set_fcs output; dl_set_fcs output
function [sdot_set_fcs, ldot_set_fcs, dl_set_fcs] = fun(l_set_fcs,vx_set_gcs,vy_set_gcs,proj_point_heading_set_gcs,proj_point_kappa_set_gcs)
% 该函数批量转化坐标得到    sdot_set_fcs, ldot_set_fcs, dl_set_fcs
% 假设最多有181个点需要转换坐标
n = 181;
% 输出初始化
sdot_set_fcs = ones(n,1)*nan; ldot_set_fcs = ones(n,1)*nan; dl_set_fcs = ones(n,1)*nan;

for i = 1:length(vx_set_gcs)
    if isnan(vx_set_gcs(i))
        break;
    end
    vector_vh = [vx_set_gcs(i),vy_set_gcs(i)];
    vector_tp = [cos(proj_point_heading_set_gcs(i)),sin(proj_point_heading_set_gcs(i))];
    vector_np = [-sin(proj_point_heading_set_gcs(i)),cos(proj_point_heading_set_gcs(i))];
    sdot_set_fcs(i) = (dot(vector_vh,vector_tp)) / (1-proj_point_kappa_set_gcs(i)*l_set_fcs(i));
    ldot_set_fcs(i) = dot(vector_vh,vector_np);
    if abs(sdot_set_fcs(i)) < 1e-6
        dl_set_fcs(i) = 0;
    else
        dl_set_fcs(i) = ldot_set_fcs(i) / sdot_set_fcs(i);
    end
end
end

== matlab function EMPlanner_cs_old/Audi_A8_Sedan_1/decision&planning module/EM Planner/Cartesian2Frenet/MATLAB Function2 ==
  data: ax_set_gcs input; sdotdot_set_fcs output; ay_set_gcs input; proj_point_heading_set_gcs input; proj_point_kappa_set_gcs input; l_set_fcs input; sdot_set_fcs input; dl_set_fcs input; ldotdot_set_fcs output; ddl_set_fcs output
function [sdotdot_set_fcs, ldotdot_set_fcs, ddl_set_fcs] = fun(ax_set_gcs,ay_set_gcs,proj_point_heading_set_gcs,proj_point_kappa_set_gcs,...
    l_set_fcs, sdot_set_fcs,dl_set_fcs)
% 该函数批量转化坐标得到    sdotdot_set_fcs, ldotdot_set_fcs, ddl_set_fcs
% 假设最多有181个点需要转换坐标
n = 181;
% 输出初始化
sdotdot_set_fcs = ones(n,1)*nan; ldotdot_set_fcs = ones(n,1)*nan; ddl_set_fcs = ones(n,1)*nan;

for i = 1:length(ax_set_gcs)
    if isnan(ax_set_gcs(i))
        break;
    end
    vector_ah = [ax_set_gcs(i),ay_set_gcs(i)];
    vector_tp = [cos(proj_point_heading_set_gcs(i)),sin(proj_point_heading_set_gcs(i))];
    vector_np = [-sin(proj_point_heading_set_gcs(i)),cos(proj_point_heading_set_gcs(i))];
    sdotdot_set_fcs(i) = (dot(vector_ah,vector_tp) + 2*proj_point_kappa_set_gcs(i)*dl_set_fcs(i)*sdot_set_fcs(i)^2) / (1-proj_point_kappa_set_gcs(i)*l_set_fcs(i));
    ldotdot_set_fcs(i) = dot(vector_ah,vector_np) - proj_point_kappa_set_gcs(i) * (1-proj_point_kappa_set_gcs(i)*l_set_fcs(i)) * sdot_set_fcs(i)^2;
    if abs(sdotdot_set_fcs(i)) < 1e-6
        ddl_set_fcs(i) = 0;
    else
        ddl_set_fcs(i) = (ldotdot_set_fcs(i) - dl_set_fcs(i) * sdotdot_set_fcs(i)) / sdot_set_fcs(i)^2;
    end
end
end

== matlab function EMPlanner_cs_old/Audi_A8_Sedan_1/decision&planning module/EM Planner/obs/obs filter ==
  data: host_x_gcs input; obs_x_set_final_gcs output; host_y_gcs input; host_heading_gcs input; obs_x_set_gcs input; obs_y_set_gcs input; obs_velocity_set_gcs input; obs_velocity_heading_set_gcs input; obs_y_set_final_gcs output; obs_velocity_set_final_gcs output; obs_velocity_heading_set_final_gcs output
function [obs_x_set_final_gcs,obs_y_set_final_gcs,obs_velocity_set_final_gcs,obs_velocity_heading_set_final_gcs] = ...
    fcn(host_x_gcs,host_y_gcs,host_heading_gcs,obs_x_set_gcs,obs_y_set_gcs,obs_velocity_set_gcs,obs_velocity_heading_set_gcs)
% 该函数将筛选障碍物，纵向[-10,60] 横向[-10,10]的障碍物才会被考虑
% 该函数只是一种单车道的临时办法，考虑到多车道情况，即使障碍物距离较远也应该考虑
% EM Planner完全体是多车道并行计算的，每个车道都生成参考线然后并行计算出多条轨迹，再选择最优的轨迹作为输出

% 假设最多检测到181个障碍物
n = 181;
% 输出初始化
obs_x_set_final_gcs = ones(n,1)*nan; obs_y_set_final_gcs = ones(n,1)*nan;
obs_velocity_set_final_gcs = ones(n,1)*nan; obs_velocity_heading_set_final_gcs = ones(n,1)*nan;

count = 1; % 记录符合要求障碍物个数
for i = 1:length(obs_x_set_gcs)
    if isnan(obs_x_set_gcs(i))
        break;
    end
%     纵向[-10,60] 是指车辆到障碍物  如果向量写反的 就会变成后方60m 前方10m 不符合原理
%     vector_host_obs = [host_x_gcs,host_y_gcs] - [obs_x_set_gcs(i),obs_y_set_gcs(i)];
    vector_host_obs = [obs_x_set_gcs(i),obs_y_set_gcs(i)] - [host_x_gcs,host_y_gcs];
    vector_th = [cos(host_heading_gcs),sin(host_heading_gcs)];
    vector_nh = [-sin(host_heading_gcs),cos(host_heading_gcs)];
    long_er = dot(vector_host_obs,vector_th);
    lat_er = dot(vector_host_obs,vector_nh);
    if long_er >= -10 && long_er <= 60 && abs(lat_er) <= 10
        obs_x_set_final_gcs(count) = obs_x_set_gcs(i);
        obs_y_set_final_gcs(count) = obs_y_set_gcs(i);
        obs_velocity_set_final_gcs(count) = obs_velocity_set_gcs(i);
        obs_velocity_heading_set_final_gcs(count) = obs_velocity_heading_set_gcs(i);
        count = count + 1;
    end
end
end

== matlab function EMPlanner_cs_old/Audi_A8_Sedan_1/decision&planning module/EM Planner/obs/Cartesian2Frenet1/MATLAB Function1 ==
  data: l_set input; s_dot_set output; vx_set input; vy_set input; proj_heading_set input; proj_kappa_set input; l_dot_set output; dl_set output
function [s_dot_set,l_dot_set,dl_set] = fcn(l_set,vx_set,vy_set,proj_heading_set,proj_kappa_set)
%该函数将计算frenet坐标系下的s_dot, l_dot, dl/ds
n = 128;
% 输出初始化
s_dot_set = ones(n,1)*nan;
l_dot_set = ones(n,1)*nan;
dl_set = ones(n,1)*nan;

for i = 1 : length(l_set)
    if isnan(l_set(i))
        break;
    end
    v_h = [vx_set(i);vy_set(i)];
    n_r = [-sin(proj_heading_set(i));cos(proj_heading_set(i))];
    t_r = [cos(proj_heading_set(i));sin(proj_heading_set(i))];
    l_dot_set(i) = v_h'*n_r;
    s_dot_set(i) = v_h'*t_r/(1 - proj_kappa_set(i)*l_set(i));
    %%%向量法做cartesian与frenet的转换要更简单，但是也有缺点，向量法必须依赖速度加速度
    %l' = l_dot/s_dot 但是如果s_dot = 0 此方法就失效了
    if abs(s_dot_set(i)) < 1e-6
        dl_set(i) = 0;
    else
        dl_set(i) = l_dot_set(i)/s_dot_set(i);
    end
end

== matlab function EMPlanner_cs_old/Audi_A8_Sedan_1/decision&planning module/EM Planner/obs/Cartesian2Frenet1/MATLAB Function2 ==
  data: ax_set input; s_dot2_set output; ay_set input; proj_heading_set input; proj_kappa_set input; l_set input; s_dot_set input; dl_set input; l_dot2_set output; ddl_set output
function [s_dot2_set,l_dot2_set,ddl_set] = fcn(ax_set,ay_set,proj_heading_set,proj_kappa_set,l_set,s_dot_set,dl_set)
%由于不知道有多少个点需要做坐标转换，设一个最大值做缓冲
n = 128;
% 输出初始化
s_dot2_set = ones(n,1)*nan;
l_dot2_set = ones(n,1)*nan;
ddl_set = ones(n,1)*nan;

for i = 1:length(l_set)
    if isnan(l_set(i))
       break;
    end
    a_h = [ax_set(i);ay_set(i)];
    n_r = [-sin(proj_heading_set(i));cos(proj_heading_set(i))];
    t_r = [cos(proj_heading_set(i));sin(proj_heading_set(i)];
    %近似认为dkr/ds 为0 简化计算
    l_dot2_set(i) = a_h'*n_r - proj_kappa_set(i) * (1 - proj_kappa_set(i) * l_set(i)) * s_dot_set(i)^2;
    s_dot2_set(i) = (1/(1 - proj_kappa_set(i) * l_set(i)))* (a_h' * t_r + 2 * proj_kappa_set(i) * dl_set(i) * s_dot_set(i)^2);
    % 要考虑加速度为0的情况
    if (s_dot2_set(i) < 1e-6)
        ddl_set(i) = 0;
    else
        ddl_set(i) = (l_dot2_set(i) - dl_set(i)*s_dot2_set(i))/(s_dot_set(i)^2);
    end
end

== matlab function EMPlanner_cs_old/Audi_A8_Sedan_1/decision&planning module/EM Planner/obs/MATLAB Function ==
  data: obs_x_set_gcs input; static_obs_x_set_gcs output; obs_y_set_gcs input; obs_velocity_set_gcs input; obs_velocity_heading_set_gcs input; static_obs_y_set_gcs output; dynamic_obs_x_set_gcs output; dynamic_obs_y_set_gcs output; dynamic_obs_vx_set_gcs output; dynamic_obs_vy_set_gcs output
function [static_obs_x_set_gcs,static_obs_y_set_gcs,dynamic_obs_x_set_gcs,dynamic_obs_y_set_gcs,...
    dynamic_obs_vx_set_gcs,dynamic_obs_vy_set_gcs] = fcn(obs_x_set_gcs,obs_y_set_gcs,obs_velocity_set_gcs,obs_velocity_heading_set_gcs)

% 该函数将分类静态障碍物和动态障碍物
% 输出初始化
n = 181;
static_obs_x_set_gcs = ones(n,1)*nan; static_obs_y_set_gcs = ones(n,1)*nan;
dynamic_obs_x_set_gcs = ones(n,1)*nan; dynamic_obs_y_set_gcs = ones(n,1)*nan;
dynamic_obs_vx_set_gcs = ones(n,1)*nan; dynamic_obs_vy_set_gcs = ones(n,1)*nan;
count_static = 1;
count_dynamic = 1;

for i = 1:length(obs_x_set_gcs)
    if isnan(obs_x_set_gcs(i))
        break;
    end
    if abs(obs_velocity_set_gcs(i)) < 0.1
        % 速度小于0.1m/s 视为静态障碍物
        static_obs_x_set_gcs(count_static) = obs_x_set_gcs(i);
        static_obs_y_set_gcs(count_static) = obs_y_set_gcs(i);
        count_static = count_static + 1;
    else
        dynamic_obs_x_set_gcs(count_dynamic) = obs_x_set_gcs(i);
        dynamic_obs_y_set_gcs(count_dynamic) = obs_y_set_gcs(i);
        dynamic_obs_vx_set_gcs(count_dynamic) = obs_velocity_set_gcs(i) * cos(obs_velocity_heading_set_gcs(i));
        dynamic_obs_vy_set_gcs(count_dynamic) = obs_velocity_set_gcs(i) * sin(obs_velocity_heading_set_gcs(i));
        count_dynamic = count_dynamic + 1;
    end
end
end

== matlab function EMPlanner_cs_old/Audi_A8_Sedan_1/全局路径(routine导航)模块/solve heading and kappa求解给定path的heading角和曲率 ==
  data: path_x_set_gcs output; path_y_set_gcs output; path_heading_set_gcs output; path_x_set_gcs input; path_y_set_gcs input; path_kappa_set_gcs output
function [path_x_set_gcs,path_y_set_gcs,path_heading_set_gcs,path_kappa_set_gcs] = fcn(path_x_set_gcs,path_y_set_gcs)
%该函数将计算全局路径的切线方向与x轴的夹角和曲率
%输入：path_x_set_gcs,path_y_set_gcs 给定路径坐标 都是列向量
%输出：path_heading_gcs path_kappa_gcs 给定路径的heading和曲率
%输出初始化
if isrow(path_x_set_gcs)
    path_x_set_gcs = path_x_set_gcs';   % 保证为列向量
    path_y_set_gcs = path_y_set_gcs';
end
[path_heading_set_gcs,path_kappa_set_gcs] = CalHeadingAndKappa(path_x_set_gcs,path_y_set_gcs);
end

== matlab function EMPlanner_cs_old/Audi_A8_Sedan_1/decision&planning module/EM Planner/calc path length and map between point and s ==
  data: path_x_set_gcs input; path_length output; path_y_set_gcs input; path_s_set_fcs output
function [path_length,path_s_set_fcs] = fcn(path_x_set_gcs,path_y_set_gcs)
% 该函数将用来计算给定路径的整个弧长 以及给定路径每个采样点到第一个采样点的弧长
n = length(path_x_set_gcs);
path_s_set_fcs = zeros(n,1);
flag = 1;
for i = 2:length(path_x_set_gcs)
    if isnan(path_x_set_gcs(i))
        flag = 0;
        break;
    end
    dis = sqrt((path_x_set_gcs(i)-path_x_set_gcs(i-1))^2 + (path_y_set_gcs(i)-path_y_set_gcs(i-1))^2);
    path_s_set_fcs(i) = path_s_set_fcs(i-1) + dis;
end

% 计算整个弧长 需要判断是遍历完推出 还是中途遇到不存在的点退出
if flag == 1
    % 正常退出
    path_length = path_s_set_fcs(end);
else
    path_length = path_s_set_fcs(i-1);
end
end
